simulink model "Week2_Problem1"  (R2020b)
settings: Solver=VariableStepAuto  StartTime=0.0  StopTime=10.0  RelTol=1e-3
settings Model: Creator=hp  LastModifiedBy=hp

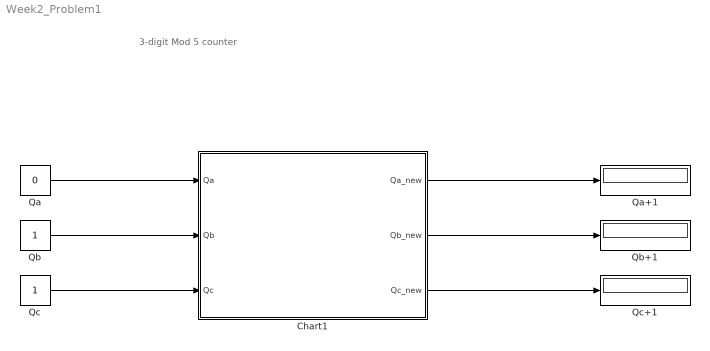
== system Week2_Problem1 ==
  note: 3-digit Mod 5 counter
  Chart1 : Stateflow chart  TreatAsAtomicUnit=on
  Qa : Constant  Value=0
  Qa+1 : Display
  Qb : Constant
  Qb+1 : Display
  Qc : Constant
  Qc+1 : Display
  wires:
  Qb/1 -> Chart1/2(Qb)
  Qc/1 -> Chart1/3(Qc)
  Qa/1 -> Chart1/1(Qa)
  Chart1/2(Qb_new) -> Qb+1/1
  Chart1/3(Qc_new) -> Qc+1/1
  Chart1/1(Qa_new) -> Qa+1/1

== stateflow chart Week2_Problem1/Chart1 ==
  state Qa0
    (default) -> (junction 10) : % When Qa=0
        | [Qa==0]
    (junction 10) -> (junction 11) [order 1] : [Qc==0]
    (junction 11) -> (junction 13) : {Qa_new=0,Qb_new=Qb,Qc_new=1;}
    (junction 10) -> (junction 15) [order 2]
    (junction 15) -> (junction 12) [order 2] : [Qb==1]{Qa_new=1,Qb_new=0,Qc_new=0;}
    (junction 15) -> (junction 12) [order 1] : [Qb==0]{Qa_new=0,Qb_new=1,Qc_new=0;}
    (junction 13) -> (junction 12)
    (junction 12) -> (junction 14)
  state Qa1
    entry:
    Qa_new=0;
    Qb_new=Qb;
    Qc_new=Qc;
  state Qa2
    entry:
    Qa_new=0;
    Qb_new=0;
    Qc_new=0;
  (default) -> Qa0
  Qa0 -> Qa1 [order 1] : [Qa==1&&Qb==0&&Qc==0]
  Qa0 -> Qa2 [order 2] : [Qa==1]
  data: Qa input; Qb input; Qc input; Qa_new output; Qb_new output; Qc_new output
